simulink library "PTCL_lib"  (Simulink 7.5)
settings: Solver=ode45  StartTime=0.0  StopTime=10.0  RelTol=1e-3
values from neighbouring files (symbols this model uses):
  pPTCL_kw_DeltaTMAvlPwr_TAB = Simulink.Parameter    [PTCL_par.m]
  pPTCL_kw_MaxIDeltaTMAvlPwr_C = Simulink.Parameter    [PTCL_par.m]
  pPTCL_kw_MaxPIDeltaTMAvlPwr_C = Simulink.Parameter    [PTCL_par.m]
  pPTCL_kw_MinIDeltaTMAvlPwr_C = Simulink.Parameter    [PTCL_par.m]
  pPTCL_kw_MinPIDeltaTMAvlPwr_C = Simulink.Parameter    [PTCL_par.m]
  pPTCL_kw_MinTMAvailPwr_C = Simulink.Parameter    [PTCL_par.m]
  pPTCL_kw_PIActDeltaPwrThrsh_C = Simulink.Parameter    [PTCL_par.m]
  pPTCL_kw_PIActHysterDeltaPwr_C = Simulink.Parameter    [PTCL_par.m]
  pPTCL_Nm_MaxTrq_CUR = Simulink.Parameter    [PTCL_par.m]
  pPTCL_Nmps_DrvTrqLowrRateLim_C = Simulink.Parameter    [PTCL_par.m]
  pPTCL_Nmps_DrvTrqUpprRateLim_C = Simulink.Parameter    [PTCL_par.m]
  pPTCL_Nmps_RcpTrqLowrRateLim_C = Simulink.Parameter    [PTCL_par.m]
  pPTCL_Nmps_RcpTrqUpprRateLim_C = Simulink.Parameter    [PTCL_par.m]
  pPTCL_pct_DrvEffiFac_C = Simulink.Parameter    [PTCL_par.m]
  pPTCL_pct_Mot1EffLowrLim_C = Simulink.Parameter    [PTCL_par.m]
  pPTCL_pct_Mot1EffUpprLim_C = Simulink.Parameter    [PTCL_par.m]
  pPTCL_pct_RcpEffiFac_C = Simulink.Parameter    [PTCL_par.m]
  pPTCL_ratio_KI4DeltaTMAvlPwr_CUR = Simulink.Parameter    [PTCL_par.m]
  pPTCL_ratio_KP4DeltaTMAvlPwr_CUR = Simulink.Parameter    [PTCL_par.m]
  pPTCL_ratio_KwToW_M = Simulink.Parameter    [PTCL_par.m]
  pPTCL_ratio_MotSpdFiltFac_C = Simulink.Parameter    [PTCL_par.m]
  pPTCL_ratio_PwrToTrqFac_M = Simulink.Parameter    [PTCL_par.m]
  pPTCL_ratio_WToKw_M = Simulink.Parameter    [PTCL_par.m]
  pPTCL_rpm_RevLowrLim_C = Simulink.Parameter    [PTCL_par.m]
  pPTCL_rpm_RevUpprLim_C = Simulink.Parameter    [PTCL_par.m]
  pPTCL_rpm_TMSpd_TAB = Simulink.Parameter    [PTCL_par.m]
undefined symbols (not defined in the file or in its folder): p_single_Minus_M, p_single_Zero_M, pESPI_kmph_MinSpdSnsrThd_C, pMCI_m_TireDiam_C, pMCI_ratio_KmPerHrToMtrPerSec_C, pMCI_ratio_TrsmRat_C, pMCI_s_NoOfSec_C
libraries: BaseOperationLib_Browser x114, simulink x1
(part 1 of 2)
settings Model: Creator=wuaibin  LastModifiedBy=wuaibin

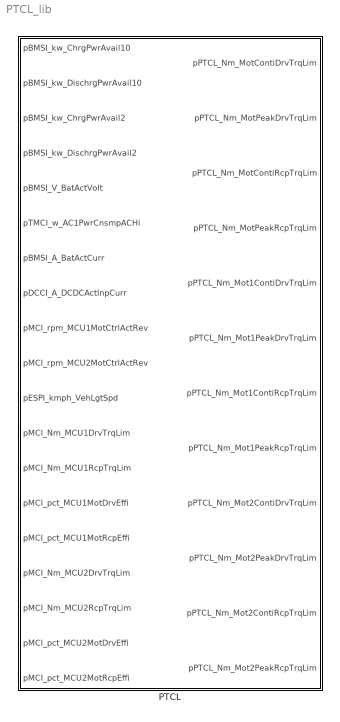
== system PTCL_lib ==
  PTCL : Subsystem  TreatAsAtomicUnit=on

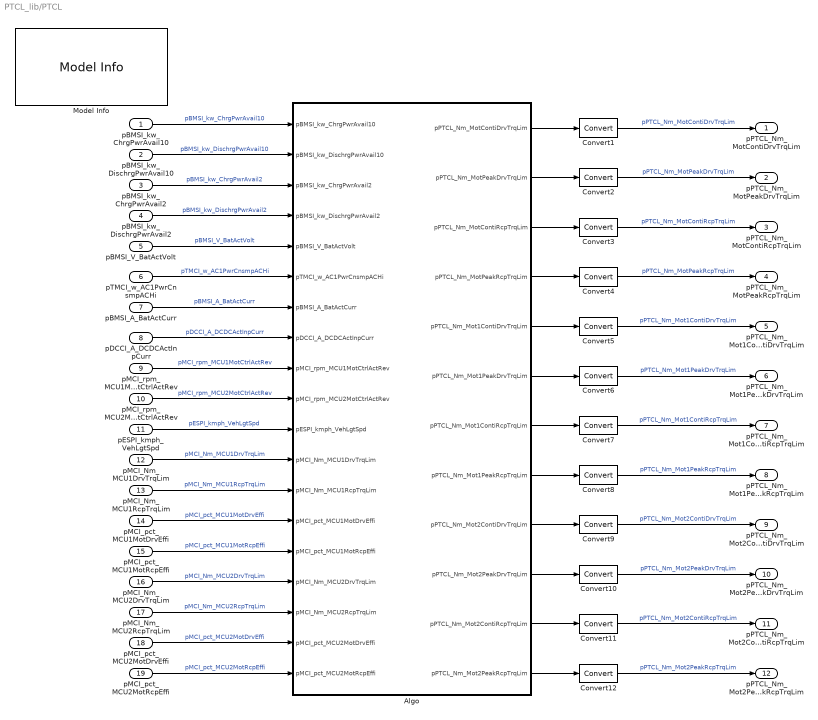
== system PTCL_lib/PTCL ==
  pBMSI_kw_ChrgPwrAvail10 : Inport
  pBMSI_kw_DischrgPwrAvail10 : Inport  Port=2
  pBMSI_kw_ChrgPwrAvail2 : Inport  Port=3
  pBMSI_kw_DischrgPwrAvail2 : Inport  Port=4
  pBMSI_V_BatActVolt : Inport  Port=5
  pTMCI_w_AC1PwrCnsmpACHi : Inport  Port=6
  pBMSI_A_BatActCurr : Inport  Port=7
  pDCCI_A_DCDCActInpCurr : Inport  Port=8
  pMCI_rpm_MCU1MotCtrlActRev : Inport  Port=9
  pMCI_rpm_MCU2MotCtrlActRev : Inport  Port=10
  pESPI_kmph_VehLgtSpd : Inport  Port=11
  pMCI_Nm_MCU1DrvTrqLim : Inport  Port=12
  pMCI_Nm_MCU1RcpTrqLim : Inport  Port=13
  pMCI_pct_MCU1MotDrvEffi : Inport  Port=14
  pMCI_pct_MCU1MotRcpEffi : Inport  Port=15
  pMCI_Nm_MCU2DrvTrqLim : Inport  Port=16
  pMCI_Nm_MCU2RcpTrqLim : Inport  Port=17
  pMCI_pct_MCU2MotDrvEffi : Inport  Port=18
  pMCI_pct_MCU2MotRcpEffi : Inport  Port=19
  Algo : Subsystem
  Convert{1..12} (12 alike) : DataTypeConversion  OutDataType=fixdt(1, 16)  OutScaling=2^0
  Model Info : simulink/Model-Wide Utilities/Model Info  SystemSampleTime=-1  InitialBlockCM=None  BlockCM=None  Frame=on  DisplayStringWithTags=Model Info\nCreated: %<Created>\nCreator: zhangqiang  HorizontalTextAlignment=Center  LeftAlignmentValue=0.5  SourceBlockDiagram=HQEV_HCU  TagMaxNumber=20
  pPTCL_Nm_MotContiDrvTrqLim : Outport
  pPTCL_Nm_MotPeakDrvTrqLim : Outport  Port=2
  pPTCL_Nm_MotContiRcpTrqLim : Outport  Port=3
  pPTCL_Nm_MotPeakRcpTrqLim : Outport  Port=4
  pPTCL_Nm_Mot1ContiDrvTrqLim : Outport  Port=5
  pPTCL_Nm_Mot1PeakDrvTrqLim : Outport  Port=6
  pPTCL_Nm_Mot1ContiRcpTrqLim : Outport  Port=7
  pPTCL_Nm_Mot1PeakRcpTrqLim : Outport  Port=8
  pPTCL_Nm_Mot2ContiDrvTrqLim : Outport  Port=9
  pPTCL_Nm_Mot2PeakDrvTrqLim : Outport  Port=10
  pPTCL_Nm_Mot2ContiRcpTrqLim : Outport  Port=11
  pPTCL_Nm_Mot2PeakRcpTrqLim : Outport  Port=12
  wires:
  pMCI_Nm_MCU2DrvTrqLim/1 -> Algo/16(pMCI_Nm_MCU2DrvTrqLim)  "pMCI_Nm_MCU2DrvTrqLim"
  pMCI_pct_MCU1MotRcpEffi/1 -> Algo/15(pMCI_pct_MCU1MotRcpEffi)  "pMCI_pct_MCU1MotRcpEffi"
  pMCI_pct_MCU1MotDrvEffi/1 -> Algo/14(pMCI_pct_MCU1MotDrvEffi)  "pMCI_pct_MCU1MotDrvEffi"
  pMCI_Nm_MCU1RcpTrqLim/1 -> Algo/13(pMCI_Nm_MCU1RcpTrqLim)  "pMCI_Nm_MCU1RcpTrqLim"
  pMCI_Nm_MCU1DrvTrqLim/1 -> Algo/12(pMCI_Nm_MCU1DrvTrqLim)  "pMCI_Nm_MCU1DrvTrqLim"
  pESPI_kmph_VehLgtSpd/1 -> Algo/11(pESPI_kmph_VehLgtSpd)  "pESPI_kmph_VehLgtSpd"
  pBMSI_kw_ChrgPwrAvail10/1 -> Algo/1(pBMSI_kw_ChrgPwrAvail10)  "pBMSI_kw_ChrgPwrAvail10"
  pBMSI_kw_DischrgPwrAvail10/1 -> Algo/2(pBMSI_kw_DischrgPwrAvail10)  "pBMSI_kw_DischrgPwrAvail10"
  pBMSI_kw_ChrgPwrAvail2/1 -> Algo/3(pBMSI_kw_ChrgPwrAvail2)  "pBMSI_kw_ChrgPwrAvail2"
  pBMSI_kw_DischrgPwrAvail2/1 -> Algo/4(pBMSI_kw_DischrgPwrAvail2)  "pBMSI_kw_DischrgPwrAvail2"
  pBMSI_V_BatActVolt/1 -> Algo/5(pBMSI_V_BatActVolt)  "pBMSI_V_BatActVolt"
  pTMCI_w_AC1PwrCnsmpACHi/1 -> Algo/6(pTMCI_w_AC1PwrCnsmpACHi)  "pTMCI_w_AC1PwrCnsmpACHi"
  pBMSI_A_BatActCurr/1 -> Algo/7(pBMSI_A_BatActCurr)  "pBMSI_A_BatActCurr"
  pDCCI_A_DCDCActInpCurr/1 -> Algo/8(pDCCI_A_DCDCActInpCurr)  "pDCCI_A_DCDCActInpCurr"
  pMCI_rpm_MCU1MotCtrlActRev/1 -> Algo/9(pMCI_rpm_MCU1MotCtrlActRev)  "pMCI_rpm_MCU1MotCtrlActRev"
  pMCI_rpm_MCU2MotCtrlActRev/1 -> Algo/10(pMCI_rpm_MCU2MotCtrlActRev)  "pMCI_rpm_MCU2MotCtrlActRev"
  Convert1/1 -> pPTCL_Nm_MotContiDrvTrqLim/1  "pPTCL_Nm_MotContiDrvTrqLim"
  Convert2/1 -> pPTCL_Nm_MotPeakDrvTrqLim/1  "pPTCL_Nm_MotPeakDrvTrqLim"
  Convert3/1 -> pPTCL_Nm_MotContiRcpTrqLim/1  "pPTCL_Nm_MotContiRcpTrqLim"
  Convert4/1 -> pPTCL_Nm_MotPeakRcpTrqLim/1  "pPTCL_Nm_MotPeakRcpTrqLim"
  Convert5/1 -> pPTCL_Nm_Mot1ContiDrvTrqLim/1  "pPTCL_Nm_Mot1ContiDrvTrqLim"
  pMCI_pct_MCU2MotRcpEffi/1 -> Algo/19(pMCI_pct_MCU2MotRcpEffi)  "pMCI_pct_MCU2MotRcpEffi"
  pMCI_pct_MCU2MotDrvEffi/1 -> Algo/18(pMCI_pct_MCU2MotDrvEffi)  "pMCI_pct_MCU2MotDrvEffi"
  pMCI_Nm_MCU2RcpTrqLim/1 -> Algo/17(pMCI_Nm_MCU2RcpTrqLim)  "pMCI_Nm_MCU2RcpTrqLim"
  Algo/1(pPTCL_Nm_MotContiDrvTrqLim) -> Convert1/1
  Algo/2(pPTCL_Nm_MotPeakDrvTrqLim) -> Convert2/1
  Algo/3(pPTCL_Nm_MotContiRcpTrqLim) -> Convert3/1
  Algo/4(pPTCL_Nm_MotPeakRcpTrqLim) -> Convert4/1
  Algo/5(pPTCL_Nm_Mot1ContiDrvTrqLim) -> Convert5/1
  Algo/6(pPTCL_Nm_Mot1PeakDrvTrqLim) -> Convert6/1
  Algo/7(pPTCL_Nm_Mot1ContiRcpTrqLim) -> Convert7/1
  Algo/8(pPTCL_Nm_Mot1PeakRcpTrqLim) -> Convert8/1
  Algo/9(pPTCL_Nm_Mot2ContiDrvTrqLim) -> Convert9/1
  Algo/10(pPTCL_Nm_Mot2PeakDrvTrqLim) -> Convert10/1
  Algo/12(pPTCL_Nm_Mot2PeakRcpTrqLim) -> Convert12/1
  Algo/11(pPTCL_Nm_Mot2ContiRcpTrqLim) -> Convert11/1
  Convert6/1 -> pPTCL_Nm_Mot1PeakDrvTrqLim/1  "pPTCL_Nm_Mot1PeakDrvTrqLim"
  Convert7/1 -> pPTCL_Nm_Mot1ContiRcpTrqLim/1  "pPTCL_Nm_Mot1ContiRcpTrqLim"
  Convert8/1 -> pPTCL_Nm_Mot1PeakRcpTrqLim/1  "pPTCL_Nm_Mot1PeakRcpTrqLim"
  Convert9/1 -> pPTCL_Nm_Mot2ContiDrvTrqLim/1  "pPTCL_Nm_Mot2ContiDrvTrqLim"
  Convert10/1 -> pPTCL_Nm_Mot2PeakDrvTrqLim/1  "pPTCL_Nm_Mot2PeakDrvTrqLim"
  Convert11/1 -> pPTCL_Nm_Mot2ContiRcpTrqLim/1  "pPTCL_Nm_Mot2ContiRcpTrqLim"
  Convert12/1 -> pPTCL_Nm_Mot2PeakRcpTrqLim/1  "pPTCL_Nm_Mot2PeakRcpTrqLim"

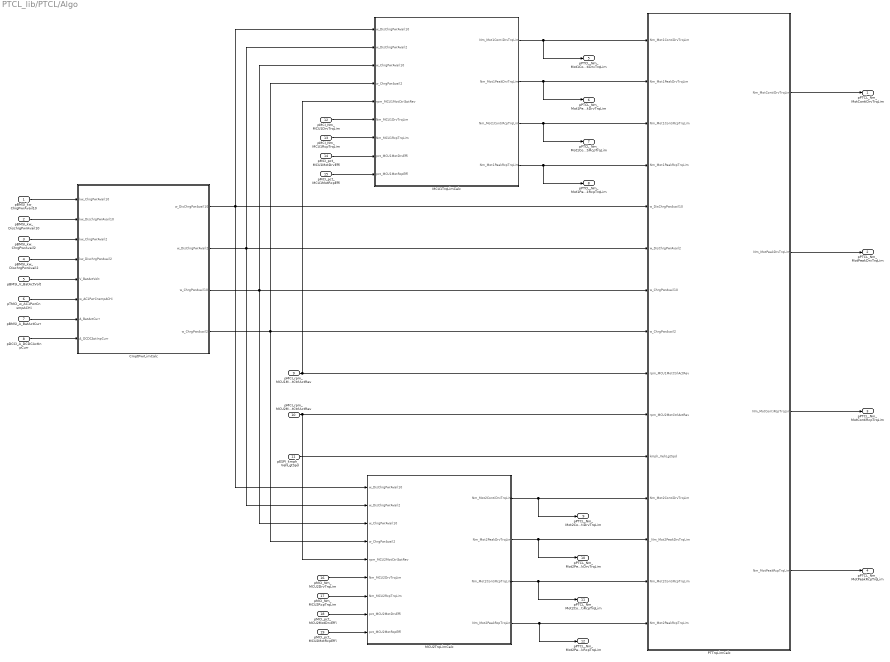
== system PTCL_lib/PTCL/Algo ==
  pBMSI_kw_ChrgPwrAvail10 : Inport
  pBMSI_kw_DischrgPwrAvail10 : Inport  Port=2
  pBMSI_kw_ChrgPwrAvail2 : Inport  Port=3
  pBMSI_kw_DischrgPwrAvail2 : Inport  Port=4
  pBMSI_V_BatActVolt : Inport  Port=5
  pTMCI_w_AC1PwrCnsmpACHi : Inport  Port=6
  pBMSI_A_BatActCurr : Inport  Port=7
  pDCCI_A_DCDCActInpCurr : Inport  Port=8
  pMCI_rpm_MCU1MotCtrlActRev : Inport  Port=9
  pMCI_rpm_MCU2MotCtrlActRev : Inport  Port=10
  pESPI_kmph_VehLgtSpd : Inport  Port=11
  pMCI_Nm_MCU1DrvTrqLim : Inport  Port=12
  pMCI_Nm_MCU1RcpTrqLim : Inport  Port=13
  pMCI_pct_MCU1MotDrvEffi : Inport  Port=14
  pMCI_pct_MCU1MotRcpEffi : Inport  Port=15
  pMCI_Nm_MCU2DrvTrqLim : Inport  Port=16
  pMCI_Nm_MCU2RcpTrqLim : Inport  Port=17
  pMCI_pct_MCU2MotDrvEffi : Inport  Port=18
  pMCI_pct_MCU2MotRcpEffi : Inport  Port=19
  CmptPwrLimCalc : Subsystem
  MCU1TrqLimCalc : Subsystem
  MCU2TrqLimCalc : Subsystem
  PTTrqLimCalc : Subsystem
  pPTCL_Nm_MotContiDrvTrqLim : Outport
  pPTCL_Nm_MotPeakDrvTrqLim : Outport  Port=2
  pPTCL_Nm_MotContiRcpTrqLim : Outport  Port=3
  pPTCL_Nm_MotPeakRcpTrqLim : Outport  Port=4
  pPTCL_Nm_Mot1ContiDrvTrqLim : Outport  Port=5
  pPTCL_Nm_Mot1PeakDrvTrqLim : Outport  Port=6
  pPTCL_Nm_Mot1ContiRcpTrqLim : Outport  Port=7
  pPTCL_Nm_Mot1PeakRcpTrqLim : Outport  Port=8
  pPTCL_Nm_Mot2ContiDrvTrqLim : Outport  Port=9
  pPTCL_Nm_Mot2PeakDrvTrqLim : Outport  Port=10
  pPTCL_Nm_Mot2ContiRcpTrqLim : Outport  Port=11
  pPTCL_Nm_Mot2PeakRcpTrqLim : Outport  Port=12
  wires:
  MCU1TrqLimCalc/1(Nm_Mot1ContiDrvTrqLim) -> pPTCL_Nm_Mot1ContiDrvTrqLim/1, PTTrqLimCalc/1(Nm_Mot1ContiDrvTrqLim)
  MCU1TrqLimCalc/2(Nm_Mot1PeakDrvTrqLim) -> pPTCL_Nm_Mot1PeakDrvTrqLim/1, PTTrqLimCalc/2(Nm_Mot1PeakDrvTrqLim)
  MCU1TrqLimCalc/3(Nm_Mot1ContiRcpTrqLim) -> pPTCL_Nm_Mot1ContiRcpTrqLim/1, PTTrqLimCalc/3(Nm_Mot1ContiRcpTrqLim)
  MCU1TrqLimCalc/4(Nm_Mot1PeakRcpTrqLim) -> pPTCL_Nm_Mot1PeakRcpTrqLim/1, PTTrqLimCalc/4(Nm_Mot1PeakRcpTrqLim)
  MCU2TrqLimCalc/1(Nm_Mot2ContiDrvTrqLim) -> PTTrqLimCalc/12(Nm_Mot2ContiDrvTrqLim), pPTCL_Nm_Mot2ContiDrvTrqLim/1
  MCU2TrqLimCalc/2(Nm_Mot2PeakDrvTrqLim) -> PTTrqLimCalc/13(_Nm_Mot2PeakDrvTrqLim), pPTCL_Nm_Mot2PeakDrvTrqLim/1
  MCU2TrqLimCalc/3(Nm_Mot2ContiRcpTrqLim) -> PTTrqLimCalc/14(Nm_Mot2ContiRcpTrqLim), pPTCL_Nm_Mot2ContiRcpTrqLim/1
  MCU2TrqLimCalc/4(Nm_Mot2PeakRcpTrqLim) -> PTTrqLimCalc/15(Nm_Mot2PeakRcpTrqLim), pPTCL_Nm_Mot2PeakRcpTrqLim/1
  PTTrqLimCalc/1(Nm_MotContiDrvTrqLim) -> pPTCL_Nm_MotContiDrvTrqLim/1
  PTTrqLimCalc/2(Nm_MotPeakDrvTrqLim) -> pPTCL_Nm_MotPeakDrvTrqLim/1
  PTTrqLimCalc/3(Nm_MotContiRcpTrqLim) -> pPTCL_Nm_MotContiRcpTrqLim/1
  PTTrqLimCalc/4(Nm_MotPeakRcpTrqLim) -> pPTCL_Nm_MotPeakRcpTrqLim/1
  CmptPwrLimCalc/1(w_DisChrgPwrAvail10) -> PTTrqLimCalc/5(w_DisChrgPwrAvail10), MCU2TrqLimCalc/1(w_DisChrgPwrAvail10), MCU1TrqLimCalc/1(w_DisChrgPwrAvail10)
  CmptPwrLimCalc/2(w_DisChrgPwrAvail2) -> PTTrqLimCalc/6(w_DisChrgPwrAvail2), MCU2TrqLimCalc/2(w_DisChrgPwrAvail2), MCU1TrqLimCalc/2(w_DisChrgPwrAvail2)
  CmptPwrLimCalc/3(w_ChrgPwrAvail10) -> PTTrqLimCalc/7(w_ChrgPwrAvail10), MCU1TrqLimCalc/3(w_ChrgPwrAvail10), MCU2TrqLimCalc/3(w_ChrgPwrAvail10)
  CmptPwrLimCalc/4(w_ChrgPwrAvail2) -> PTTrqLimCalc/8(w_ChrgPwrAvail2), MCU2TrqLimCalc/4(w_ChrgPwrAvail2), MCU1TrqLimCalc/4(w_ChrgPwrAvail2)
  pBMSI_kw_ChrgPwrAvail10/1 -> CmptPwrLimCalc/1(kw_ChrgPwrAvail10)
  pBMSI_kw_DischrgPwrAvail10/1 -> CmptPwrLimCalc/2(kw_DischrgPwrAvail10)
  pBMSI_kw_ChrgPwrAvail2/1 -> CmptPwrLimCalc/3(kw_ChrgPwrAvail2)
  pBMSI_kw_DischrgPwrAvail2/1 -> CmptPwrLimCalc/4(kw_DischrgPwrAvail2)
  pBMSI_V_BatActVolt/1 -> CmptPwrLimCalc/5(V_BatActVolt)
  pTMCI_w_AC1PwrCnsmpACHi/1 -> CmptPwrLimCalc/6(w_AC1PwrCnsmpACHi)
  pBMSI_A_BatActCurr/1 -> CmptPwrLimCalc/7(A_BatActCurr)
  pDCCI_A_DCDCActInpCurr/1 -> CmptPwrLimCalc/8(A_DCDCActInpCurr)
  pMCI_rpm_MCU1MotCtrlActRev/1 -> PTTrqLimCalc/9(rpm_MCU1MotCtrlActRev), MCU1TrqLimCalc/5(rpm_MCU1MotCtrlActRev)
  pMCI_rpm_MCU2MotCtrlActRev/1 -> PTTrqLimCalc/10(rpm_MCU2MotCtrlActRev), MCU2TrqLimCalc/5(rpm_MCU2MotCtrlActRev)
  pESPI_kmph_VehLgtSpd/1 -> PTTrqLimCalc/11(kmph_VehLgtSpd)
  pMCI_Nm_MCU1DrvTrqLim/1 -> MCU1TrqLimCalc/6(Nm_MCU1DrvTrqLim)
  pMCI_Nm_MCU1RcpTrqLim/1 -> MCU1TrqLimCalc/7(Nm_MCU1RcpTrqLim)
  pMCI_Nm_MCU2DrvTrqLim/1 -> MCU2TrqLimCalc/6(Nm_MCU2DrvTrqLim)
  pMCI_Nm_MCU2RcpTrqLim/1 -> MCU2TrqLimCalc/7(Nm_MCU2RcpTrqLim)
  pMCI_pct_MCU2MotDrvEffi/1 -> MCU2TrqLimCalc/8(pct_MCU2MotDrvEffi)
  pMCI_pct_MCU2MotRcpEffi/1 -> MCU2TrqLimCalc/9(pct_MCU2MotRcpEffi)
  pMCI_pct_MCU1MotDrvEffi/1 -> MCU1TrqLimCalc/8(pct_MCU1MotDrvEffi)
  pMCI_pct_MCU1MotRcpEffi/1 -> MCU1TrqLimCalc/9(pct_MCU1MotRcpEffi)

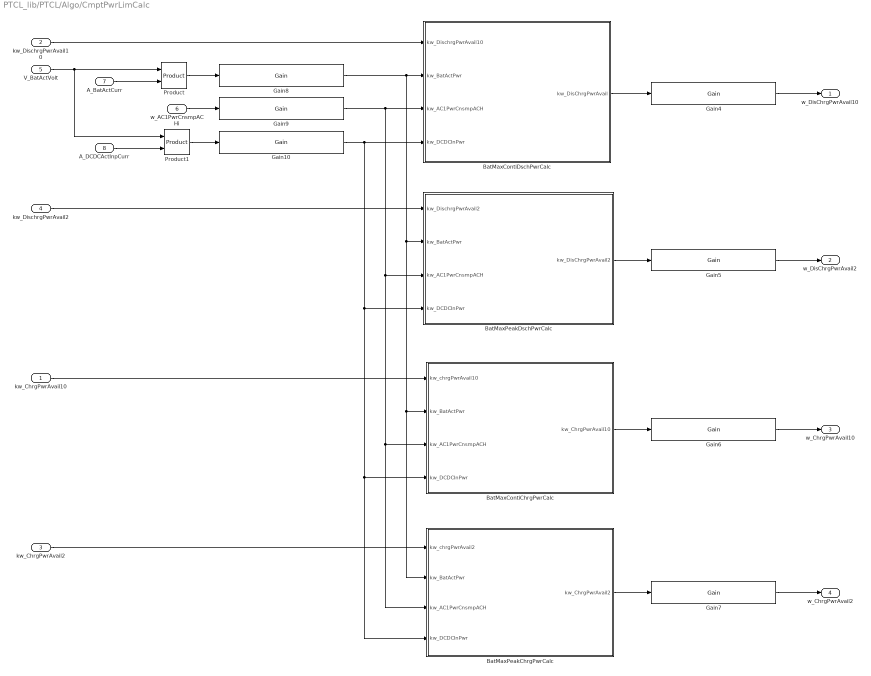
== system PTCL_lib/PTCL/Algo/CmptPwrLimCalc ==
  kw_ChrgPwrAvail10 : Inport
  kw_DischrgPwrAvail10 : Inport  Port=2
  kw_ChrgPwrAvail2 : Inport  Port=3
  kw_DischrgPwrAvail2 : Inport  Port=4
  V_BatActVolt : Inport  Port=5
  w_AC1PwrCnsmpACHi : Inport  Port=6  OutDataType=fixdt(1, 16)  OutScaling=2^0
  A_BatActCurr : Inport  Port=7
  A_DCDCActInpCurr : Inport  Port=8  OutDataType=fixdt(1, 16)  OutScaling=2^0
  BatMaxContiChrgPwrCalc : Subsystem
  BatMaxContiDschPwrCalc : Subsystem
  BatMaxPeakChrgPwrCalc : Subsystem
  BatMaxPeakDschPwrCalc : Subsystem
  Gain10 : BaseOperationLib_Browser/Math Operations Changed/Gain  Gain=pPTCL_ratio_WToKw_M  Multiplication=Element-wise(K.*u)  ParamMin=[]  ParamMax=[]  ParameterDataType=fixdt(1, 16)  ParameterScalingMode=Best Precision: Matrix-wise  ParameterScaling=2^0  ParamDataTypeStr=Inherit: Inherit from 'Gain'  OutMin=[]  OutMax=[]  OutDataType=fixdt(1, 16)  OutScaling=2^0  SaturateOnIntegerOverflow=on
  Gain{4..7} (4 alike) : BaseOperationLib_Browser/Math Operations Changed/Gain  Gain=pPTCL_ratio_KwToW_M  Multiplication=Element-wise(K.*u)  ParamMin=[]  ParamMax=[]  ParameterDataType=fixdt(1, 16)  ParameterScalingMode=Best Precision: Matrix-wise  ParameterScaling=2^0  ParamDataTypeStr=Inherit: Inherit from 'Gain'  OutMin=[]  OutMax=[]  OutDataType=fixdt(1, 16)  OutScaling=2^0  SaturateOnIntegerOverflow=on
  Gain8 : BaseOperationLib_Browser/Math Operations Changed/Gain  Gain=pPTCL_ratio_WToKw_M  Multiplication=Element-wise(K.*u)  ParamMin=[]  ParamMax=[]  ParameterDataType=fixdt(1, 16)  ParameterScalingMode=Best Precision: Matrix-wise  ParameterScaling=2^0  ParamDataTypeStr=Inherit: Inherit from 'Gain'  OutMin=[]  OutMax=[]  OutDataType=fixdt(1, 16)  OutScaling=2^0  SaturateOnIntegerOverflow=on
  Gain9 : BaseOperationLib_Browser/Math Operations Changed/Gain  Gain=pPTCL_ratio_WToKw_M  Multiplication=Element-wise(K.*u)  ParamMin=[]  ParamMax=[]  ParameterDataType=fixdt(1, 16)  ParameterScalingMode=Best Precision: Matrix-wise  ParameterScaling=2^0  ParamDataTypeStr=Inherit: Inherit from 'Gain'  OutMin=[]  OutMax=[]  OutDataType=fixdt(1, 16)  OutScaling=2^0  SaturateOnIntegerOverflow=on
  Product : BaseOperationLib_Browser/Math Operations Changed/Product  Inputs=2  Multiplication=Element-wise(.*)  OutMin=[]  OutMax=[]  OutDataType=fixdt(1,16,0)  OutScaling=[]  OutDataTypeStr=Inherit: Inherit via back propagation  RndMeth=Zero  SaturateOnIntegerOverflow=on
  Product1 : BaseOperationLib_Browser/Math Operations Changed/Product  Inputs=2  Multiplication=Element-wise(.*)  OutMin=[]  OutMax=[]  OutDataType=fixdt(1,16,0)  OutScaling=[]  OutDataTypeStr=Inherit: Inherit via back propagation  RndMeth=Zero  SaturateOnIntegerOverflow=on
  w_DisChrgPwrAvail10 : Outport  OutDataType=fixdt(1, 16)  OutScaling=2^0
  w_DisChrgPwrAvail2 : Outport  Port=2  OutDataType=fixdt(1, 16)  OutScaling=2^0
  w_ChrgPwrAvail10 : Outport  Port=3  OutDataType=fixdt(1, 16)  OutScaling=2^0
  w_ChrgPwrAvail2 : Outport  Port=4  OutDataType=fixdt(1, 16)  OutScaling=2^0
  wires:
  V_BatActVolt/1 -> Product/1, Product1/1
  A_BatActCurr/1 -> Product/2
  A_DCDCActInpCurr/1 -> Product1/2
  kw_DischrgPwrAvail10/1 -> BatMaxContiDschPwrCalc/1(kw_DischrgPwrAvail10)
  Product/1 -> Gain8/1
  w_AC1PwrCnsmpACHi/1 -> Gain9/1
  Product1/1 -> Gain10/1
  kw_DischrgPwrAvail2/1 -> BatMaxPeakDschPwrCalc/1(kw_DischrgPwrAvail2)
  kw_ChrgPwrAvail10/1 -> BatMaxContiChrgPwrCalc/1(kw_chrgPwrAvail10)
  kw_ChrgPwrAvail2/1 -> BatMaxPeakChrgPwrCalc/1(kw_chrgPwrAvail2)
  BatMaxPeakChrgPwrCalc/1(kw_ChrgPwrAvail2) -> Gain7/1
  BatMaxContiChrgPwrCalc/1(kw_ChrgPwrAvail10) -> Gain6/1
  BatMaxPeakDschPwrCalc/1(kw_DisChrgPwrAvail2) -> Gain5/1
  BatMaxContiDschPwrCalc/1(kw_DisChrgPwrAvail) -> Gain4/1
  Gain4/1 -> w_DisChrgPwrAvail10/1
  Gain5/1 -> w_DisChrgPwrAvail2/1
  Gain6/1 -> w_ChrgPwrAvail10/1
  Gain7/1 -> w_ChrgPwrAvail2/1
  Gain8/1 -> BatMaxContiDschPwrCalc/2(kw_BatActPwr), BatMaxPeakDschPwrCalc/2(kw_BatActPwr), BatMaxContiChrgPwrCalc/2(kw_BatActPwr), BatMaxPeakChrgPwrCalc/2(kw_BatActPwr)
  Gain9/1 -> BatMaxContiDschPwrCalc/3(kw_AC1PwrCnsmpACH), BatMaxPeakDschPwrCalc/3(kw_AC1PwrCnsmpACH), BatMaxContiChrgPwrCalc/3(kw_AC1PwrCnsmpACH), BatMaxPeakChrgPwrCalc/3(kw_AC1PwrCnsmpACH)
  Gain10/1 -> BatMaxContiDschPwrCalc/4(kw_DCDCInPwr), BatMaxPeakDschPwrCalc/4(kw_DCDCInPwr), BatMaxContiChrgPwrCalc/4(kw_DCDCInPwr), BatMaxPeakChrgPwrCalc/4(kw_DCDCInPwr)

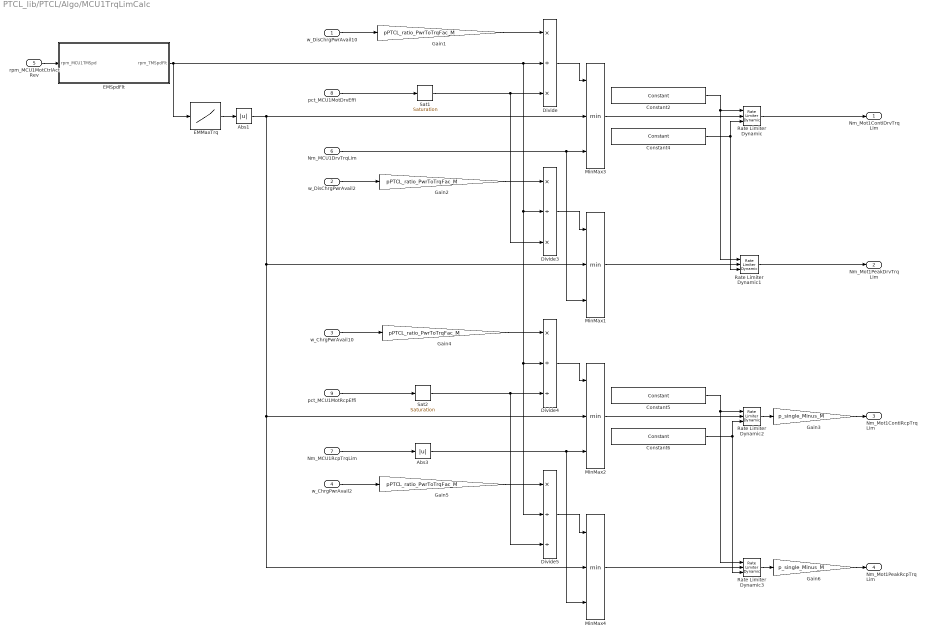
== system PTCL_lib/PTCL/Algo/MCU1TrqLimCalc ==
  w_DisChrgPwrAvail10 : Inport
  w_DisChrgPwrAvail2 : Inport  Port=2
  w_ChrgPwrAvail10 : Inport  Port=3
  w_ChrgPwrAvail2 : Inport  Port=4
  rpm_MCU1MotCtrlActRev : Inport  Port=5
  Nm_MCU1DrvTrqLim : Inport  Port=6
  Nm_MCU1RcpTrqLim : Inport  Port=7
  pct_MCU1MotDrvEffi : Inport  Port=8
  pct_MCU1MotRcpEffi : Inport  Port=9
  Abs1 : Abs  SaturateOnIntegerOverflow=on
      mask Display: patch([0 1 1 1 .75], [1 1 0 .75 1], [0 1 0]);
  Abs3 : Abs  SaturateOnIntegerOverflow=on
      mask Display: patch([0 1 1 1 .75], [1 1 0 .75 1], [0 1 0]);
  Constant2 : BaseOperationLib_Browser/Sources&Sinks/Constant  Value=pPTCL_Nmps_DrvTrqUpprRateLim_C  OutMin=[]  OutMax=[]  OutDataType=fixdt(1, 16)  ConRadixGroup=Use specified scaling  OutScaling=2^0  OutDataTypeStr=Inherit: Inherit from 'Constant value'
  Constant4 : BaseOperationLib_Browser/Sources&Sinks/Constant  Value=pPTCL_Nmps_DrvTrqLowrRateLim_C  OutMin=[]  OutMax=[]  OutDataType=fixdt(1, 16)  ConRadixGroup=Use specified scaling  OutScaling=2^0  OutDataTypeStr=Inherit: Inherit from 'Constant value'
  Constant5 : BaseOperationLib_Browser/Sources&Sinks/Constant  Value=pPTCL_Nmps_RcpTrqUpprRateLim_C  OutMin=[]  OutMax=[]  OutDataType=fixdt(1, 16)  ConRadixGroup=Use specified scaling  OutScaling=2^0  OutDataTypeStr=Inherit: Inherit from 'Constant value'
  Constant6 : BaseOperationLib_Browser/Sources&Sinks/Constant  Value=pPTCL_Nmps_RcpTrqLowrRateLim_C  OutMin=[]  OutMax=[]  OutDataType=fixdt(1, 16)  ConRadixGroup=Use specified scaling  OutScaling=2^0  OutDataTypeStr=Inherit: Inherit from 'Constant value'
  Divide : Product  Inputs=*/*  OutDataTypeStr=Inherit: Inherit via back propagation  SaturateOnIntegerOverflow=on
      mask Display: patch([0 1 1 1 .75], [1 1 0 .75 1], [0 1 0]);
  Divide3 : Product  Inputs=*/*  OutDataTypeStr=Inherit: Inherit via back propagation  SaturateOnIntegerOverflow=on
      mask Display: patch([0 1 1 1 .75], [1 1 0 .75 1], [0 1 0]);
  Divide4 : Product  Inputs=*//  OutDataTypeStr=Inherit: Inherit via back propagation  SaturateOnIntegerOverflow=on
      mask Display: patch([0 1 1 1 .75], [1 1 0 .75 1], [0 1 0]);
  Divide5 : Product  Inputs=*//  OutDataTypeStr=Inherit: Inherit via back propagation  SaturateOnIntegerOverflow=on
      mask Display: patch([0 1 1 1 .75], [1 1 0 .75 1], [0 1 0]);
  EMMaxTrq : Lookup  InputValues=pPTCL_rpm_TMSpd_TAB  Table=pPTCL_Nm_MaxTrq_CUR  LookUpMeth=Interpolation-Use End Values  OutDataTypeStr=Inherit: Inherit via back propagation  SaturateOnIntegerOverflow=on
      settings: AttributesFormatString=X:%<InputValues>\nTAB:%<Table>
      mask Display: patch([0 1 1 1 .75], [1 1 0 .75 1], [0 1 0]);
  EMSpdFlt : Subsystem
  Gain{1..2,4..5} (4 alike) : Gain  Gain=pPTCL_ratio_PwrToTrqFac_M  SaturateOnIntegerOverflow=on  OutDataTypeStr=Inherit: Same as input
      mask Display: patch([0 1 1 1 .75], [1 1 0 .75 1], [0 1 0]);
  Gain3 : Gain  Gain=p_single_Minus_M  SaturateOnIntegerOverflow=on  OutDataTypeStr=Inherit: Same as input
      mask Display: patch([0 1 1 1 .75], [1 1 0 .75 1], [0 1 0]);
  Gain6 : Gain  Gain=p_single_Minus_M  SaturateOnIntegerOverflow=on  OutDataTypeStr=Inherit: Same as input
      mask Display: patch([0 1 1 1 .75], [1 1 0 .75 1], [0 1 0]);
  MinMax{1..4} (4 alike) : MinMax  Inputs=3  SaturateOnIntegerOverflow=on  InputSameDT=on
      mask Display: patch([0 1 1 1 .75], [1 1 0 .75 1], [0 1 0]);
  Rate Limiter Dynamic{,1..3} (4 alike) : BaseOperationLib_Browser/Discontinuities Unchanged/Rate Limiter Dynamic  SystemSampleTime=-1
  Sat1 : BaseOperationLib_Browser/Discontinuities Unchanged/Saturation  UpperLimit=pPTCL_pct_Mot1EffUpprLim_C  LowerLimit=pPTCL_pct_Mot1EffLowrLim_C  OutMin=[]  OutMax=[]  OutDataType=fixdt(1, 16)  OutScaling=2^0  OutDataTypeStr=Inherit: Inherit via back propagation
      settings: AttributesFormatString=ULim:%<UpperLimit>\nLLim:%<LowerLimit>
  Sat2 : BaseOperationLib_Browser/Discontinuities Unchanged/Saturation  UpperLimit=pPTCL_pct_Mot1EffUpprLim_C  LowerLimit=pPTCL_pct_Mot1EffLowrLim_C  OutMin=[]  OutMax=[]  OutDataType=fixdt(1, 16)  OutScaling=2^0  OutDataTypeStr=Inherit: Inherit via back propagation
      settings: AttributesFormatString=ULim:%<UpperLimit>\nLLim:%<LowerLimit>
  Nm_Mot1ContiDrvTrqLim : Outport
  Nm_Mot1PeakDrvTrqLim : Outport  Port=2
  Nm_Mot1ContiRcpTrqLim : Outport  Port=3
  Nm_Mot1PeakRcpTrqLim : Outport  Port=4
  wires:
  Abs3/1 -> MinMax4/3, MinMax2/3
  Nm_MCU1DrvTrqLim/1 -> MinMax1/3, MinMax3/3
  Nm_MCU1RcpTrqLim/1 -> Abs3/1
  Abs1/1 -> MinMax4/2, MinMax2/2, MinMax1/2, MinMax3/2
  EMMaxTrq/1 -> Abs1/1
  w_DisChrgPwrAvail10/1 -> Gain1/1
  rpm_MCU1MotCtrlActRev/1 -> EMSpdFlt/1(rpm_MCU1TMSpd)
  Divide/1 -> MinMax3/1
  Sat1/1 -> Divide/3, Divide3/3
  pct_MCU1MotDrvEffi/1 -> Sat1/1
  Gain1/1 -> Divide/1
  w_DisChrgPwrAvail2/1 -> Gain2/1
  Gain2/1 -> Divide3/1
  Divide3/1 -> MinMax1/1
  w_ChrgPwrAvail10/1 -> Gain4/1
  Divide4/1 -> MinMax2/1
  pct_MCU1MotRcpEffi/1 -> Sat2/1
  Gain4/1 -> Divide4/1
  w_ChrgPwrAvail2/1 -> Gain5/1
  Gain5/1 -> Divide5/1
  Divide5/1 -> MinMax4/1
  EMSpdFlt/1(rpm_TMSpdFlt) -> Divide/2, Divide4/2, Divide5/2, Divide3/2, EMMaxTrq/1
  Rate Limiter Dynamic/1 -> Nm_Mot1ContiDrvTrqLim/1
  MinMax3/1 -> Rate Limiter Dynamic/2
  Rate Limiter Dynamic1/1 -> Nm_Mot1PeakDrvTrqLim/1
  MinMax1/1 -> Rate Limiter Dynamic1/2
  Rate Limiter Dynamic2/1 -> Gain3/1
  Rate Limiter Dynamic3/1 -> Gain6/1
  Constant2/1 -> Rate Limiter Dynamic/1, Rate Limiter Dynamic1/1
  Constant4/1 -> Rate Limiter Dynamic/3, Rate Limiter Dynamic1/3
  Constant5/1 -> Rate Limiter Dynamic2/1, Rate Limiter Dynamic3/1
  Constant6/1 -> Rate Limiter Dynamic2/3, Rate Limiter Dynamic3/3
  MinMax2/1 -> Rate Limiter Dynamic2/2
  MinMax4/1 -> Rate Limiter Dynamic3/2
  Gain3/1 -> Nm_Mot1ContiRcpTrqLim/1
  Gain6/1 -> Nm_Mot1PeakRcpTrqLim/1
  Sat2/1 -> Divide5/3, Divide4/3

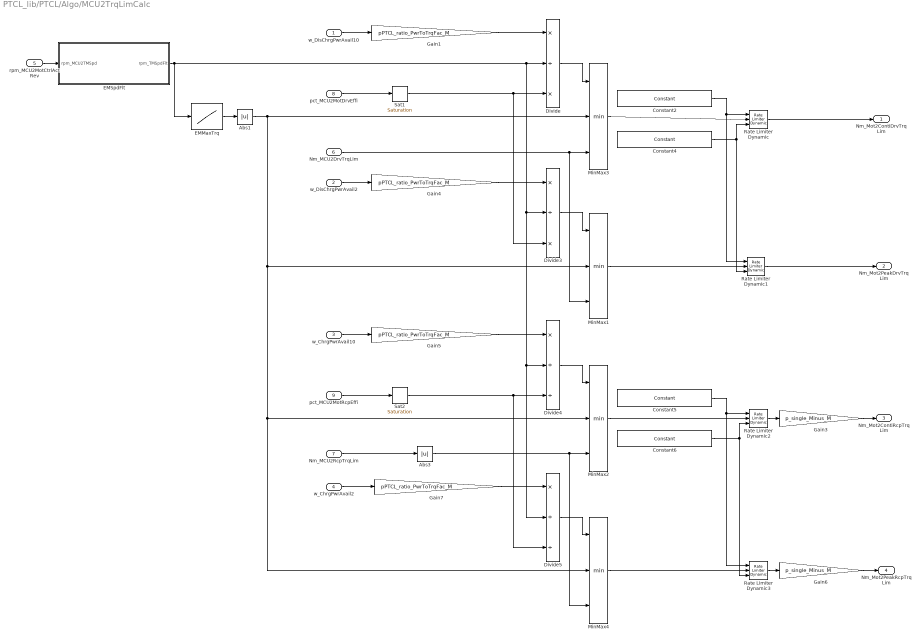
== system PTCL_lib/PTCL/Algo/MCU2TrqLimCalc ==
  w_DisChrgPwrAvail10 : Inport
  w_DisChrgPwrAvail2 : Inport  Port=2
  w_ChrgPwrAvail10 : Inport  Port=3
  w_ChrgPwrAvail2 : Inport  Port=4
  rpm_MCU2MotCtrlActRev : Inport  Port=5
  Nm_MCU2DrvTrqLim : Inport  Port=6
  Nm_MCU2RcpTrqLim : Inport  Port=7
  pct_MCU2MotDrvEffi : Inport  Port=8
  pct_MCU2MotRcpEffi : Inport  Port=9
  Abs1 : Abs  SaturateOnIntegerOverflow=on
      mask Display: patch([0 1 1 1 .75], [1 1 0 .75 1], [0 1 0]);
  Abs3 : Abs  SaturateOnIntegerOverflow=on
      mask Display: patch([0 1 1 1 .75], [1 1 0 .75 1], [0 1 0]);
  Constant2 : BaseOperationLib_Browser/Sources&Sinks/Constant  Value=pPTCL_Nmps_DrvTrqUpprRateLim_C  OutMin=[]  OutMax=[]  OutDataType=fixdt(1, 16)  ConRadixGroup=Use specified scaling  OutScaling=2^0  OutDataTypeStr=Inherit: Inherit from 'Constant value'
  Constant4 : BaseOperationLib_Browser/Sources&Sinks/Constant  Value=pPTCL_Nmps_DrvTrqLowrRateLim_C  OutMin=[]  OutMax=[]  OutDataType=fixdt(1, 16)  ConRadixGroup=Use specified scaling  OutScaling=2^0  OutDataTypeStr=Inherit: Inherit from 'Constant value'
  Constant5 : BaseOperationLib_Browser/Sources&Sinks/Constant  Value=pPTCL_Nmps_RcpTrqUpprRateLim_C  OutMin=[]  OutMax=[]  OutDataType=fixdt(1, 16)  ConRadixGroup=Use specified scaling  OutScaling=2^0  OutDataTypeStr=Inherit: Inherit from 'Constant value'
  Constant6 : BaseOperationLib_Browser/Sources&Sinks/Constant  Value=pPTCL_Nmps_RcpTrqLowrRateLim_C  OutMin=[]  OutMax=[]  OutDataType=fixdt(1, 16)  ConRadixGroup=Use specified scaling  OutScaling=2^0  OutDataTypeStr=Inherit: Inherit from 'Constant value'
  Divide : Product  Inputs=*/*  OutDataTypeStr=Inherit: Inherit via back propagation  SaturateOnIntegerOverflow=on
      mask Display: patch([0 1 1 1 .75], [1 1 0 .75 1], [0 1 0]);
  Divide3 : Product  Inputs=*/*  OutDataTypeStr=Inherit: Inherit via back propagation  SaturateOnIntegerOverflow=on
      mask Display: patch([0 1 1 1 .75], [1 1 0 .75 1], [0 1 0]);
  Divide4 : Product  Inputs=*//  OutDataTypeStr=Inherit: Inherit via back propagation  SaturateOnIntegerOverflow=on
      mask Display: patch([0 1 1 1 .75], [1 1 0 .75 1], [0 1 0]);
  Divide5 : Product  Inputs=*//  OutDataTypeStr=Inherit: Inherit via back propagation  SaturateOnIntegerOverflow=on
      mask Display: patch([0 1 1 1 .75], [1 1 0 .75 1], [0 1 0]);
  EMMaxTrq : Lookup  InputValues=pPTCL_rpm_TMSpd_TAB  Table=pPTCL_Nm_MaxTrq_CUR  LookUpMeth=Interpolation-Use End Values  OutDataTypeStr=Inherit: Inherit via back propagation  SaturateOnIntegerOverflow=on
      settings: AttributesFormatString=X:%<InputValues>\nTAB:%<Table>
      mask Display: patch([0 1 1 1 .75], [1 1 0 .75 1], [0 1 0]);
  EMSpdFlt : Subsystem
  Gain{1,4..5,7} (4 alike) : Gain  Gain=pPTCL_ratio_PwrToTrqFac_M  SaturateOnIntegerOverflow=on  OutDataTypeStr=Inherit: Same as input
      mask Display: patch([0 1 1 1 .75], [1 1 0 .75 1], [0 1 0]);
  Gain3 : Gain  Gain=p_single_Minus_M  SaturateOnIntegerOverflow=on  OutDataTypeStr=Inherit: Same as input
      mask Display: patch([0 1 1 1 .75], [1 1 0 .75 1], [0 1 0]);
  Gain6 : Gain  Gain=p_single_Minus_M  SaturateOnIntegerOverflow=on  OutDataTypeStr=Inherit: Same as input
      mask Display: patch([0 1 1 1 .75], [1 1 0 .75 1], [0 1 0]);
  MinMax{1..4} (4 alike) : MinMax  Inputs=3  SaturateOnIntegerOverflow=on  InputSameDT=on
      mask Display: patch([0 1 1 1 .75], [1 1 0 .75 1], [0 1 0]);
  Rate Limiter Dynamic{,1..3} (4 alike) : BaseOperationLib_Browser/Discontinuities Unchanged/Rate Limiter Dynamic  SystemSampleTime=-1
  Sat1 : BaseOperationLib_Browser/Discontinuities Unchanged/Saturation  UpperLimit=pPTCL_pct_Mot1EffUpprLim_C  LowerLimit=pPTCL_pct_Mot1EffLowrLim_C  OutMin=[]  OutMax=[]  OutDataType=fixdt(1, 16)  OutScaling=2^0  OutDataTypeStr=Inherit: Inherit via back propagation
      settings: AttributesFormatString=ULim:%<UpperLimit>\nLLim:%<LowerLimit>
  Sat2 : BaseOperationLib_Browser/Discontinuities Unchanged/Saturation  UpperLimit=pPTCL_pct_Mot1EffUpprLim_C  LowerLimit=pPTCL_pct_Mot1EffLowrLim_C  OutMin=[]  OutMax=[]  OutDataType=fixdt(1, 16)  OutScaling=2^0  OutDataTypeStr=Inherit: Inherit via back propagation
      settings: AttributesFormatString=ULim:%<UpperLimit>\nLLim:%<LowerLimit>
  Nm_Mot2ContiDrvTrqLim : Outport
  Nm_Mot2PeakDrvTrqLim : Outport  Port=2
  Nm_Mot2ContiRcpTrqLim : Outport  Port=3
  Nm_Mot2PeakRcpTrqLim : Outport  Port=4
  wires:
  EMSpdFlt/1(rpm_TMSpdFlt) -> EMMaxTrq/1, Divide3/2, Divide5/2, Divide4/2, Divide/2
  Divide5/1 -> MinMax4/1
  Gain7/1 -> Divide5/1
  w_ChrgPwrAvail2/1 -> Gain7/1
  Gain5/1 -> Divide4/1
  pct_MCU2MotRcpEffi/1 -> Sat2/1
  Sat2/1 -> Divide4/3, Divide5/3
  Divide4/1 -> MinMax2/1
  w_ChrgPwrAvail10/1 -> Gain5/1
  Divide3/1 -> MinMax1/1
  Gain4/1 -> Divide3/1
  w_DisChrgPwrAvail2/1 -> Gain4/1
  Gain1/1 -> Divide/1
  pct_MCU2MotDrvEffi/1 -> Sat1/1
  Sat1/1 -> Divide3/3, Divide/3
  Divide/1 -> MinMax3/1
  rpm_MCU2MotCtrlActRev/1 -> EMSpdFlt/1(rpm_MCU2TMSpd)
  w_DisChrgPwrAvail10/1 -> Gain1/1
  EMMaxTrq/1 -> Abs1/1
  Abs1/1 -> MinMax3/2, MinMax1/2, MinMax2/2, MinMax4/2
  Nm_MCU2RcpTrqLim/1 -> Abs3/1
  Nm_MCU2DrvTrqLim/1 -> MinMax3/3, MinMax1/3
  Abs3/1 -> MinMax2/3, MinMax4/3
  Rate Limiter Dynamic/1 -> Nm_Mot2ContiDrvTrqLim/1
  MinMax3/1 -> Rate Limiter Dynamic/2
  Rate Limiter Dynamic1/1 -> Nm_Mot2PeakDrvTrqLim/1
  MinMax1/1 -> Rate Limiter Dynamic1/2
  Rate Limiter Dynamic2/1 -> Gain3/1
  MinMax2/1 -> Rate Limiter Dynamic2/2
  Rate Limiter Dynamic3/1 -> Gain6/1
  MinMax4/1 -> Rate Limiter Dynamic3/2
  Constant2/1 -> Rate Limiter Dynamic/1, Rate Limiter Dynamic1/1
  Constant4/1 -> Rate Limiter Dynamic/3, Rate Limiter Dynamic1/3
  Constant5/1 -> Rate Limiter Dynamic2/1, Rate Limiter Dynamic3/1
  Constant6/1 -> Rate Limiter Dynamic2/3, Rate Limiter Dynamic3/3
  Gain3/1 -> Nm_Mot2ContiRcpTrqLim/1
  Gain6/1 -> Nm_Mot2PeakRcpTrqLim/1

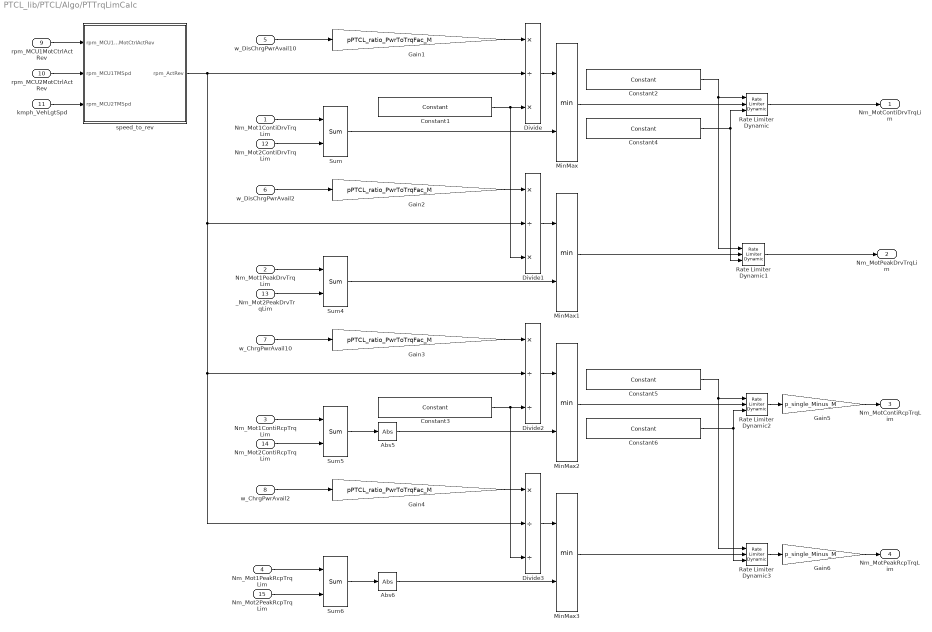
== system PTCL_lib/PTCL/Algo/PTTrqLimCalc ==
  Nm_Mot1ContiDrvTrqLim : Inport
  Nm_Mot1PeakDrvTrqLim : Inport  Port=2
  Nm_Mot1ContiRcpTrqLim : Inport  Port=3
  Nm_Mot1PeakRcpTrqLim : Inport  Port=4
  w_DisChrgPwrAvail10 : Inport  Port=5
  w_DisChrgPwrAvail2 : Inport  Port=6
  w_ChrgPwrAvail10 : Inport  Port=7
  w_ChrgPwrAvail2 : Inport  Port=8
  rpm_MCU1MotCtrlActRev : Inport  Port=9  OutDataType=fixdt(1, 16)  OutScaling=2^0
  rpm_MCU2MotCtrlActRev : Inport  Port=10  OutDataType=fixdt(1, 16)  OutScaling=2^0
  kmph_VehLgtSpd : Inport  Port=11  OutDataType=fixdt(1, 16)  OutScaling=2^0
  Nm_Mot2ContiDrvTrqLim : Inport  Port=12
  _Nm_Mot2PeakDrvTrqLim : Inport  Port=13
  Nm_Mot2ContiRcpTrqLim : Inport  Port=14
  Nm_Mot2PeakRcpTrqLim : Inport  Port=15
  Abs5 : BaseOperationLib_Browser/Math Operations Changed/Abs  OutMax=[]  OutDataType=fixdt(1, 16)  OutScaling=2^0
  Abs6 : BaseOperationLib_Browser/Math Operations Changed/Abs  OutMax=[]  OutDataType=fixdt(1, 16)  OutScaling=2^0
  Constant1 : BaseOperationLib_Browser/Sources&Sinks/Constant  Value=pPTCL_pct_DrvEffiFac_C  OutMin=[]  OutMax=[]  OutDataType=fixdt(1, 16)  ConRadixGroup=Use specified scaling  OutScaling=2^0  OutDataTypeStr=Inherit: Inherit from 'Constant value'
  Constant2 : BaseOperationLib_Browser/Sources&Sinks/Constant  Value=pPTCL_Nmps_DrvTrqUpprRateLim_C  OutMin=[]  OutMax=[]  OutDataType=fixdt(1, 16)  ConRadixGroup=Use specified scaling  OutScaling=2^0  OutDataTypeStr=Inherit: Inherit from 'Constant value'
  Constant3 : BaseOperationLib_Browser/Sources&Sinks/Constant  Value=pPTCL_pct_RcpEffiFac_C  OutMin=[]  OutMax=[]  OutDataType=fixdt(1, 16)  ConRadixGroup=Use specified scaling  OutScaling=2^0  OutDataTypeStr=Inherit: Inherit from 'Constant value'
  Constant4 : BaseOperationLib_Browser/Sources&Sinks/Constant  Value=pPTCL_Nmps_DrvTrqLowrRateLim_C  OutMin=[]  OutMax=[]  OutDataType=fixdt(1, 16)  ConRadixGroup=Use specified scaling  OutScaling=2^0  OutDataTypeStr=Inherit: Inherit from 'Constant value'
  Constant5 : BaseOperationLib_Browser/Sources&Sinks/Constant  Value=pPTCL_Nmps_RcpTrqUpprRateLim_C  OutMin=[]  OutMax=[]  OutDataType=fixdt(1, 16)  ConRadixGroup=Use specified scaling  OutScaling=2^0  OutDataTypeStr=Inherit: Inherit from 'Constant value'
  Constant6 : BaseOperationLib_Browser/Sources&Sinks/Constant  Value=pPTCL_Nmps_RcpTrqLowrRateLim_C  OutMin=[]  OutMax=[]  OutDataType=fixdt(1, 16)  ConRadixGroup=Use specified scaling  OutScaling=2^0  OutDataTypeStr=Inherit: Inherit from 'Constant value'
  Divide : Product  Inputs=*/*  OutDataTypeStr=Inherit: Inherit via back propagation  SaturateOnIntegerOverflow=on
      mask Display: patch([0 1 1 1 .75], [1 1 0 .75 1], [0 1 0]);
  Divide1 : Product  Inputs=*/*  OutDataTypeStr=Inherit: Inherit via back propagation  SaturateOnIntegerOverflow=on
      mask Display: patch([0 1 1 1 .75], [1 1 0 .75 1], [0 1 0]);
  Divide2 : Product  Inputs=*//  OutDataTypeStr=Inherit: Inherit via back propagation  SaturateOnIntegerOverflow=on
      mask Display: patch([0 1 1 1 .75], [1 1 0 .75 1], [0 1 0]);
  Divide3 : Product  Inputs=*//  OutDataTypeStr=Inherit: Inherit via back propagation  SaturateOnIntegerOverflow=on
      mask Display: patch([0 1 1 1 .75], [1 1 0 .75 1], [0 1 0]);
  Gain{1..4} (4 alike) : Gain  Gain=pPTCL_ratio_PwrToTrqFac_M  SaturateOnIntegerOverflow=on  OutDataTypeStr=Inherit: Same as input
      mask Display: patch([0 1 1 1 .75], [1 1 0 .75 1], [0 1 0]);
  Gain5 : Gain  Gain=p_single_Minus_M  SaturateOnIntegerOverflow=on  OutDataTypeStr=Inherit: Same as input
      mask Display: patch([0 1 1 1 .75], [1 1 0 .75 1], [0 1 0]);
  Gain6 : Gain  Gain=p_single_Minus_M  SaturateOnIntegerOverflow=on  OutDataTypeStr=Inherit: Same as input
      mask Display: patch([0 1 1 1 .75], [1 1 0 .75 1], [0 1 0]);
  MinMax{,1..3} (4 alike) : MinMax  Inputs=2  SaturateOnIntegerOverflow=on  InputSameDT=on
      mask Display: patch([0 1 1 1 .75], [1 1 0 .75 1], [0 1 0]);
  Rate Limiter Dynamic{,1..3} (4 alike) : BaseOperationLib_Browser/Discontinuities Unchanged/Rate Limiter Dynamic  SystemSampleTime=-1
  Sum{,4..6} (4 alike) : BaseOperationLib_Browser/Math Operations Changed/Sum  Inputs=++  InputSameDT=on  OutMin=[]  OutMax=[]  OutDataType=fixdt(1, 16)  OutScaling=2^0  SaturateOnIntegerOverflow=on
  speed_to_rev : Subsystem
  Nm_MotContiDrvTrqLim : Outport
  Nm_MotPeakDrvTrqLim : Outport  Port=2
  Nm_MotContiRcpTrqLim : Outport  Port=3
  Nm_MotPeakRcpTrqLim : Outport  Port=4
  wires:
  Rate Limiter Dynamic/1 -> Nm_MotContiDrvTrqLim/1
  w_DisChrgPwrAvail10/1 -> Gain1/1
  Divide/1 -> MinMax/1
  Constant1/1 -> Divide/3, Divide1/3
  Gain1/1 -> Divide/1
  Sum/1 -> MinMax/2
  Nm_Mot1ContiDrvTrqLim/1 -> Sum/1
  Nm_Mot2ContiDrvTrqLim/1 -> Sum/2
  w_DisChrgPwrAvail2/1 -> Gain2/1
  w_ChrgPwrAvail10/1 -> Gain3/1
  speed_to_rev/1(rpm_ActRev) -> Divide3/2, Divide2/2, Divide1/2, Divide/2
  Divide1/1 -> MinMax1/1
  Gain2/1 -> Divide1/1
  Sum4/1 -> MinMax1/2
  Divide2/1 -> MinMax2/1
  Gain3/1 -> Divide2/1
  Sum5/1 -> Abs5/1
  Divide3/1 -> MinMax3/1
  Gain4/1 -> Divide3/1
  Sum6/1 -> Abs6/1
  Nm_Mot1PeakDrvTrqLim/1 -> Sum4/1
  _Nm_Mot2PeakDrvTrqLim/1 -> Sum4/2
  Nm_Mot1PeakRcpTrqLim/1 -> Sum6/1
  Nm_Mot2PeakRcpTrqLim/1 -> Sum6/2
  Nm_Mot1ContiRcpTrqLim/1 -> Sum5/1
  Nm_Mot2ContiRcpTrqLim/1 -> Sum5/2
  w_ChrgPwrAvail2/1 -> Gain4/1
  MinMax/1 -> Rate Limiter Dynamic/2
  Rate Limiter Dynamic1/1 -> Nm_MotPeakDrvTrqLim/1
  MinMax1/1 -> Rate Limiter Dynamic1/2
  Rate Limiter Dynamic2/1 -> Gain5/1
  MinMax2/1 -> Rate Limiter Dynamic2/2
  Rate Limiter Dynamic3/1 -> Gain6/1
  MinMax3/1 -> Rate Limiter Dynamic3/2
  rpm_MCU1MotCtrlActRev/1 -> speed_to_rev/1(rpm_MCU1MotCtrlActRev)
  rpm_MCU2MotCtrlActRev/1 -> speed_to_rev/2(rpm_MCU1TMSpd)
  kmph_VehLgtSpd/1 -> speed_to_rev/3(rpm_MCU2TMSpd)
  Abs5/1 -> MinMax2/2
  Abs6/1 -> MinMax3/2
  Constant3/1 -> Divide2/3, Divide3/3
  Constant2/1 -> Rate Limiter Dynamic/1, Rate Limiter Dynamic1/1
  Constant4/1 -> Rate Limiter Dynamic/3, Rate Limiter Dynamic1/3
  Constant5/1 -> Rate Limiter Dynamic2/1, Rate Limiter Dynamic3/1
  Constant6/1 -> Rate Limiter Dynamic2/3, Rate Limiter Dynamic3/3
  Gain5/1 -> Nm_MotContiRcpTrqLim/1
  Gain6/1 -> Nm_MotPeakRcpTrqLim/1

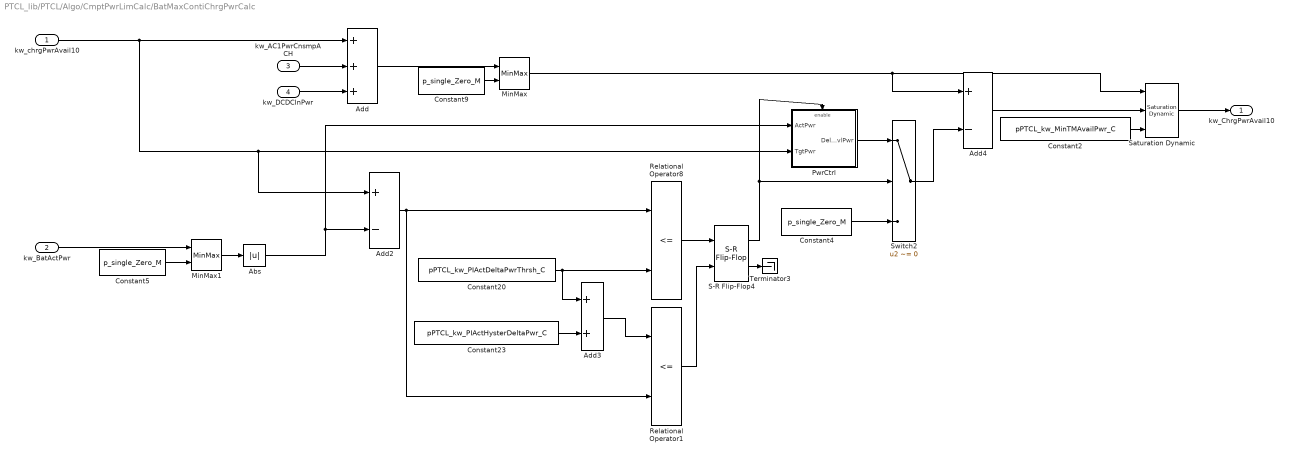
== system PTCL_lib/PTCL/Algo/CmptPwrLimCalc/BatMaxContiChrgPwrCalc ==
  kw_chrgPwrAvail10 : Inport
  kw_BatActPwr : Inport  Port=2
  kw_AC1PwrCnsmpACH : Inport  Port=3
  kw_DCDCInPwr : Inport  Port=4
  Abs : Abs  SaturateOnIntegerOverflow=on
      mask Display: patch([0 1 1 1 .75], [1 1 0 .75 1], [0 1 0]);
  Add : Sum  Inputs=+++  SaturateOnIntegerOverflow=on  InputSameDT=on  OutDataTypeStr=Inherit: Same as first input
      mask Display: patch([0 1 1 1 .75], [1 1 0 .75 1], [0 1 0]);
  Add2 : Sum  Inputs=+-  SaturateOnIntegerOverflow=on  InputSameDT=on  OutDataTypeStr=Inherit: Same as first input
      mask Display: patch([0 1 1 1 .75], [1 1 0 .75 1], [0 1 0]);
  Add3 : Sum  SaturateOnIntegerOverflow=on  InputSameDT=on  OutDataTypeStr=Inherit: Same as first input
      mask Display: patch([0 1 1 1 .75], [1 1 0 .75 1], [0 1 0]);
  Add4 : Sum  Inputs=+-  SaturateOnIntegerOverflow=on  InputSameDT=on  OutDataTypeStr=Inherit: Same as first input
      mask Display: patch([0 1 1 1 .75], [1 1 0 .75 1], [0 1 0]);
  Constant2 : Constant  Value=pPTCL_kw_MinTMAvailPwr_C
      mask Display: patch([0 1 1 1 .75], [1 1 0 .75 1], [0 1 0]);
  Constant20 : Constant  Value=pPTCL_kw_PIActDeltaPwrThrsh_C
      mask Display: patch([0 1 1 1 .75], [1 1 0 .75 1], [0 1 0]);
  Constant23 : Constant  Value=pPTCL_kw_PIActHysterDeltaPwr_C
      mask Display: patch([0 1 1 1 .75], [1 1 0 .75 1], [0 1 0]);
  Constant4 : Constant  Value=p_single_Zero_M
      mask Display: patch([0 1 1 1 .75], [1 1 0 .75 1], [0 1 0]);
  Constant5 : Constant  Value=p_single_Zero_M
      mask Display: patch([0 1 1 1 .75], [1 1 0 .75 1], [0 1 0]);
  Constant9 : Constant  Value=p_single_Zero_M
      mask Display: patch([0 1 1 1 .75], [1 1 0 .75 1], [0 1 0]);
  MinMax : BaseOperationLib_Browser/Math Operations Changed/MinMax  Function=max  Inputs=2  InputSameDT=on  OutMin=[]  OutMax=[]  OutDataType=fixdt(1,16,0)  OutScaling=[]  SaturateOnIntegerOverflow=on
  MinMax1 : BaseOperationLib_Browser/Math Operations Changed/MinMax  Function=min  Inputs=2  InputSameDT=on  OutMin=[]  OutMax=[]  OutDataType=fixdt(1,16,0)  OutScaling=[]  SaturateOnIntegerOverflow=on
  PwrCtrl : Subsystem
  Relational Operator1 : RelationalOperator  Operator=<=  LogicOutDataTypeMode=Specify via dialog  LogicDataType=PDT_Bool  OutDataTypeStr=PDT_Bool  InputSameDT=on
      mask Display: patch([0 1 1 1 .75], [1 1 0 .75 1], [0 1 0]);
  Relational Operator8 : RelationalOperator  Operator=<=  LogicOutDataTypeMode=Specify via dialog  LogicDataType=PDT_Bool  OutDataTypeStr=PDT_Bool  InputSameDT=on
      mask Display: patch([0 1 1 1 .75], [1 1 0 .75 1], [0 1 0]);
  S-R Flip-Flop4 : BaseOperationLib_Browser/Others Unchanged/S-R Flip-Flop  SystemSampleTime=-1  initial_condition=0
  Saturation Dynamic : BaseOperationLib_Browser/Discontinuities Unchanged/Saturation Dynamic  SystemSampleTime=-1  OutMin=[]  OutMax=[]  OutDataTypeStr=Inherit: Same as second input  OutDataType=fixdt(1, 16)  OutScaling=2^-10  DoSatur=on
  Switch2 : Switch  Criteria=u2 ~= 0  SaturateOnIntegerOverflow=on  InputSameDT=on
      mask Display: patch([0 1 1 1 .75], [1 1 0 .75 1], [0 1 0]);
  Terminator3 : Terminator
  kw_ChrgPwrAvail10 : Outport  OutDataType=fixdt(1, 16)  OutScaling=2^0
  wires:
  kw_BatActPwr/1 -> MinMax1/1
  MinMax1/1 -> Abs/1
  Constant5/1 -> MinMax1/2
  Abs/1 -> Add2/2, PwrCtrl/1(ActPwr)
  Add/1 -> MinMax/1
  Constant9/1 -> MinMax/2
  Constant2/1 -> Saturation Dynamic/3
  kw_chrgPwrAvail10/1 -> Add/1, Add2/1, PwrCtrl/2(TgtPwr)
  S-R Flip-Flop4/2 -> Terminator3/1
  Add2/1 -> Relational Operator8/1, Relational Operator1/2
  Constant20/1 -> Relational Operator8/2, Add3/1
  Constant23/1 -> Add3/2
  Add3/1 -> Relational Operator1/1
  Relational Operator8/1 -> S-R Flip-Flop4/1
  Relational Operator1/1 -> S-R Flip-Flop4/2
  S-R Flip-Flop4/1 -> Switch2/2, PwrCtrl/Enable
  Constant4/1 -> Switch2/3
  Switch2/1 -> Add4/2
  PwrCtrl/1(DeltaEMAvlPwr) -> Switch2/1
  Add4/1 -> Saturation Dynamic/2
  MinMax/1 -> Add4/1, Saturation Dynamic/1
  kw_AC1PwrCnsmpACH/1 -> Add/2
  kw_DCDCInPwr/1 -> Add/3
  Saturation Dynamic/1 -> kw_ChrgPwrAvail10/1

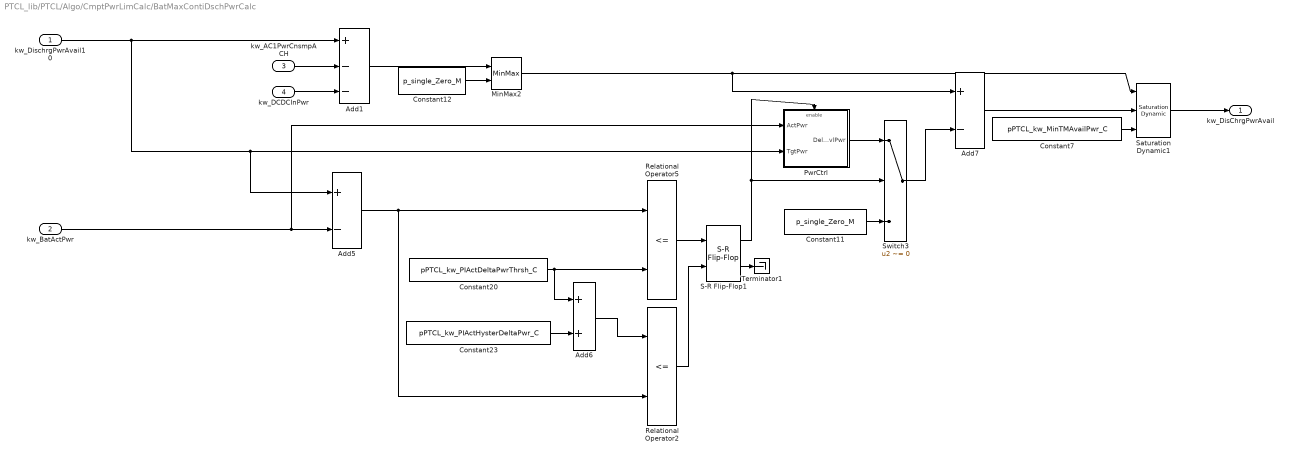
== system PTCL_lib/PTCL/Algo/CmptPwrLimCalc/BatMaxContiDschPwrCalc ==
  kw_DischrgPwrAvail10 : Inport
  kw_BatActPwr : Inport  Port=2
  kw_AC1PwrCnsmpACH : Inport  Port=3
  kw_DCDCInPwr : Inport  Port=4
  Add1 : Sum  Inputs=+--  SaturateOnIntegerOverflow=on  InputSameDT=on  OutDataTypeStr=Inherit: Same as first input
      mask Display: patch([0 1 1 1 .75], [1 1 0 .75 1], [0 1 0]);
  Add5 : Sum  Inputs=+-  SaturateOnIntegerOverflow=on  InputSameDT=on  OutDataTypeStr=Inherit: Same as first input
      mask Display: patch([0 1 1 1 .75], [1 1 0 .75 1], [0 1 0]);
  Add6 : Sum  SaturateOnIntegerOverflow=on  InputSameDT=on  OutDataTypeStr=Inherit: Same as first input
      mask Display: patch([0 1 1 1 .75], [1 1 0 .75 1], [0 1 0]);
  Add7 : Sum  Inputs=+-  SaturateOnIntegerOverflow=on  InputSameDT=on  OutDataTypeStr=Inherit: Same as first input
      mask Display: patch([0 1 1 1 .75], [1 1 0 .75 1], [0 1 0]);
  Constant11 : Constant  Value=p_single_Zero_M
      mask Display: patch([0 1 1 1 .75], [1 1 0 .75 1], [0 1 0]);
  Constant12 : Constant  Value=p_single_Zero_M
      mask Display: patch([0 1 1 1 .75], [1 1 0 .75 1], [0 1 0]);
  Constant20 : Constant  Value=pPTCL_kw_PIActDeltaPwrThrsh_C
      mask Display: patch([0 1 1 1 .75], [1 1 0 .75 1], [0 1 0]);
  Constant23 : Constant  Value=pPTCL_kw_PIActHysterDeltaPwr_C
      mask Display: patch([0 1 1 1 .75], [1 1 0 .75 1], [0 1 0]);
  Constant7 : Constant  Value=pPTCL_kw_MinTMAvailPwr_C
      mask Display: patch([0 1 1 1 .75], [1 1 0 .75 1], [0 1 0]);
  MinMax2 : BaseOperationLib_Browser/Math Operations Changed/MinMax  Function=max  Inputs=2  InputSameDT=on  OutMin=[]  OutMax=[]  OutDataType=fixdt(1,16,0)  OutScaling=[]  SaturateOnIntegerOverflow=on
  PwrCtrl : Subsystem
  Relational Operator2 : RelationalOperator  Operator=<=  LogicOutDataTypeMode=Specify via dialog  LogicDataType=PDT_Bool  OutDataTypeStr=PDT_Bool  InputSameDT=on
      mask Display: patch([0 1 1 1 .75], [1 1 0 .75 1], [0 1 0]);
  Relational Operator5 : RelationalOperator  Operator=<=  LogicOutDataTypeMode=Specify via dialog  LogicDataType=PDT_Bool  OutDataTypeStr=PDT_Bool  InputSameDT=on
      mask Display: patch([0 1 1 1 .75], [1 1 0 .75 1], [0 1 0]);
  S-R Flip-Flop1 : BaseOperationLib_Browser/Others Unchanged/S-R Flip-Flop  SystemSampleTime=-1  initial_condition=0
  Saturation Dynamic1 : BaseOperationLib_Browser/Discontinuities Unchanged/Saturation Dynamic  SystemSampleTime=-1  OutMin=[]  OutMax=[]  OutDataTypeStr=Inherit: Same as second input  OutDataType=fixdt(1, 16)  OutScaling=2^-10  DoSatur=on
  Switch3 : Switch  Criteria=u2 ~= 0  SaturateOnIntegerOverflow=on  InputSameDT=on
      mask Display: patch([0 1 1 1 .75], [1 1 0 .75 1], [0 1 0]);
  Terminator1 : Terminator
  kw_DisChrgPwrAvail : Outport  OutDataType=fixdt(1, 16)  OutScaling=2^0
  wires:
  Add1/1 -> MinMax2/1
  Constant12/1 -> MinMax2/2
  Constant7/1 -> Saturation Dynamic1/3
  kw_DischrgPwrAvail10/1 -> Add1/1, Add5/1, PwrCtrl/2(TgtPwr)
  S-R Flip-Flop1/2 -> Terminator1/1
  Add5/1 -> Relational Operator5/1, Relational Operator2/2
  Constant20/1 -> Relational Operator5/2, Add6/1
  Constant23/1 -> Add6/2
  Add6/1 -> Relational Operator2/1
  Relational Operator5/1 -> S-R Flip-Flop1/1
  Relational Operator2/1 -> S-R Flip-Flop1/2
  S-R Flip-Flop1/1 -> Switch3/2, PwrCtrl/Enable
  Constant11/1 -> Switch3/3
  Switch3/1 -> Add7/2
  PwrCtrl/1(DeltaEMAvlPwr) -> Switch3/1
  Add7/1 -> Saturation Dynamic1/2
  MinMax2/1 -> Add7/1, Saturation Dynamic1/1
  kw_BatActPwr/1 -> Add5/2, PwrCtrl/1(ActPwr)
  kw_AC1PwrCnsmpACH/1 -> Add1/2
  kw_DCDCInPwr/1 -> Add1/3
  Saturation Dynamic1/1 -> kw_DisChrgPwrAvail/1

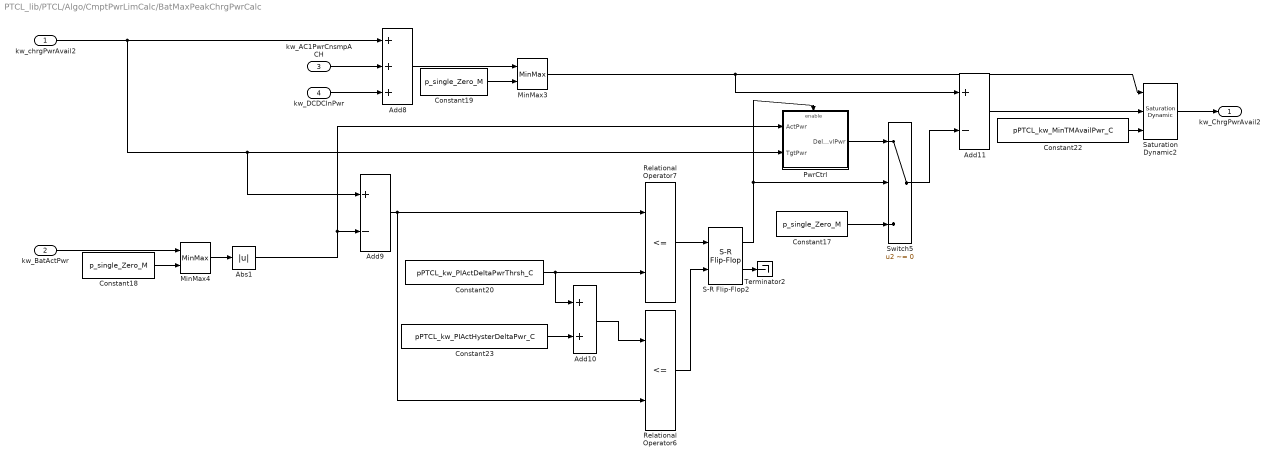
== system PTCL_lib/PTCL/Algo/CmptPwrLimCalc/BatMaxPeakChrgPwrCalc ==
  kw_chrgPwrAvail2 : Inport
  kw_BatActPwr : Inport  Port=2
  kw_AC1PwrCnsmpACH : Inport  Port=3
  kw_DCDCInPwr : Inport  Port=4
  Abs1 : Abs  SaturateOnIntegerOverflow=on
      mask Display: patch([0 1 1 1 .75], [1 1 0 .75 1], [0 1 0]);
  Add10 : Sum  SaturateOnIntegerOverflow=on  InputSameDT=on  OutDataTypeStr=Inherit: Same as first input
      mask Display: patch([0 1 1 1 .75], [1 1 0 .75 1], [0 1 0]);
  Add11 : Sum  Inputs=+-  SaturateOnIntegerOverflow=on  InputSameDT=on  OutDataTypeStr=Inherit: Same as first input
      mask Display: patch([0 1 1 1 .75], [1 1 0 .75 1], [0 1 0]);
  Add8 : Sum  Inputs=+++  SaturateOnIntegerOverflow=on  InputSameDT=on  OutDataTypeStr=Inherit: Same as first input
      mask Display: patch([0 1 1 1 .75], [1 1 0 .75 1], [0 1 0]);
  Add9 : Sum  Inputs=+-  SaturateOnIntegerOverflow=on  InputSameDT=on  OutDataTypeStr=Inherit: Same as first input
      mask Display: patch([0 1 1 1 .75], [1 1 0 .75 1], [0 1 0]);
  Constant17 : Constant  Value=p_single_Zero_M
      mask Display: patch([0 1 1 1 .75], [1 1 0 .75 1], [0 1 0]);
  Constant18 : Constant  Value=p_single_Zero_M
      mask Display: patch([0 1 1 1 .75], [1 1 0 .75 1], [0 1 0]);
  Constant19 : Constant  Value=p_single_Zero_M
      mask Display: patch([0 1 1 1 .75], [1 1 0 .75 1], [0 1 0]);
  Constant20 : Constant  Value=pPTCL_kw_PIActDeltaPwrThrsh_C
      mask Display: patch([0 1 1 1 .75], [1 1 0 .75 1], [0 1 0]);
  Constant22 : Constant  Value=pPTCL_kw_MinTMAvailPwr_C
      mask Display: patch([0 1 1 1 .75], [1 1 0 .75 1], [0 1 0]);
  Constant23 : Constant  Value=pPTCL_kw_PIActHysterDeltaPwr_C
      mask Display: patch([0 1 1 1 .75], [1 1 0 .75 1], [0 1 0]);
  MinMax3 : BaseOperationLib_Browser/Math Operations Changed/MinMax  Function=max  Inputs=2  InputSameDT=on  OutMin=[]  OutMax=[]  OutDataType=fixdt(1,16,0)  OutScaling=[]  SaturateOnIntegerOverflow=on
  MinMax4 : BaseOperationLib_Browser/Math Operations Changed/MinMax  Function=min  Inputs=2  InputSameDT=on  OutMin=[]  OutMax=[]  OutDataType=fixdt(1,16,0)  OutScaling=[]  SaturateOnIntegerOverflow=on
  PwrCtrl : Subsystem
  Relational Operator6 : RelationalOperator  Operator=<=  LogicOutDataTypeMode=Specify via dialog  LogicDataType=PDT_Bool  OutDataTypeStr=PDT_Bool  InputSameDT=on
      mask Display: patch([0 1 1 1 .75], [1 1 0 .75 1], [0 1 0]);
  Relational Operator7 : RelationalOperator  Operator=<=  LogicOutDataTypeMode=Specify via dialog  LogicDataType=PDT_Bool  OutDataTypeStr=PDT_Bool  InputSameDT=on
      mask Display: patch([0 1 1 1 .75], [1 1 0 .75 1], [0 1 0]);
  S-R Flip-Flop2 : BaseOperationLib_Browser/Others Unchanged/S-R Flip-Flop  SystemSampleTime=-1  initial_condition=0
  Saturation Dynamic2 : BaseOperationLib_Browser/Discontinuities Unchanged/Saturation Dynamic  SystemSampleTime=-1  OutMin=[]  OutMax=[]  OutDataTypeStr=Inherit: Same as second input  OutDataType=fixdt(1, 16)  OutScaling=2^-10  DoSatur=on
  Switch5 : Switch  Criteria=u2 ~= 0  SaturateOnIntegerOverflow=on  InputSameDT=on
      mask Display: patch([0 1 1 1 .75], [1 1 0 .75 1], [0 1 0]);
  Terminator2 : Terminator
  kw_ChrgPwrAvail2 : Outport  OutDataType=fixdt(1, 16)  OutScaling=2^0
  wires:
  MinMax3/1 -> Saturation Dynamic2/1, Add11/1
  Add11/1 -> Saturation Dynamic2/2
  PwrCtrl/1(DeltaEMAvlPwr) -> Switch5/1
  Switch5/1 -> Add11/2
  Constant17/1 -> Switch5/3
  S-R Flip-Flop2/1 -> Switch5/2, PwrCtrl/Enable
  Relational Operator6/1 -> S-R Flip-Flop2/2
  Relational Operator7/1 -> S-R Flip-Flop2/1
  Add10/1 -> Relational Operator6/1
  Constant23/1 -> Add10/2
  Constant20/1 -> Add10/1, Relational Operator7/2
  Add9/1 -> Relational Operator6/2, Relational Operator7/1
  S-R Flip-Flop2/2 -> Terminator2/1
  kw_chrgPwrAvail2/1 -> Add8/1, Add9/1, PwrCtrl/2(TgtPwr)
  Constant22/1 -> Saturation Dynamic2/3
  Constant19/1 -> MinMax3/2
  Add8/1 -> MinMax3/1
  Abs1/1 -> Add9/2, PwrCtrl/1(ActPwr)
  Constant18/1 -> MinMax4/2
  MinMax4/1 -> Abs1/1
  kw_BatActPwr/1 -> MinMax4/1
  kw_AC1PwrCnsmpACH/1 -> Add8/2
  kw_DCDCInPwr/1 -> Add8/3
  Saturation Dynamic2/1 -> kw_ChrgPwrAvail2/1

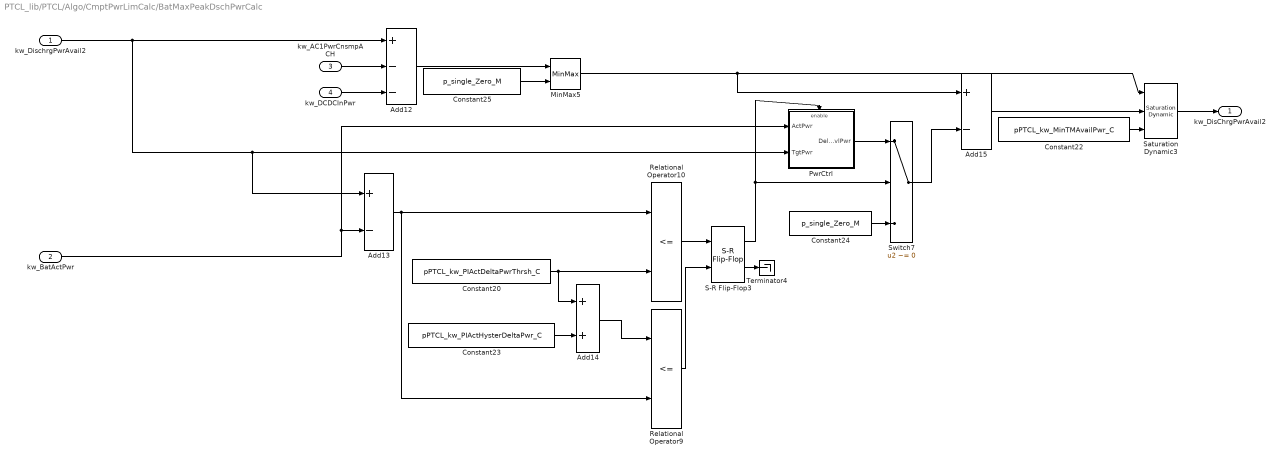
== system PTCL_lib/PTCL/Algo/CmptPwrLimCalc/BatMaxPeakDschPwrCalc ==
  kw_DischrgPwrAvail2 : Inport
  kw_BatActPwr : Inport  Port=2
  kw_AC1PwrCnsmpACH : Inport  Port=3
  kw_DCDCInPwr : Inport  Port=4
  Add12 : Sum  Inputs=+--  SaturateOnIntegerOverflow=on  InputSameDT=on  OutDataTypeStr=Inherit: Same as first input
      mask Display: patch([0 1 1 1 .75], [1 1 0 .75 1], [0 1 0]);
  Add13 : Sum  Inputs=+-  SaturateOnIntegerOverflow=on  InputSameDT=on  OutDataTypeStr=Inherit: Same as first input
      mask Display: patch([0 1 1 1 .75], [1 1 0 .75 1], [0 1 0]);
  Add14 : Sum  SaturateOnIntegerOverflow=on  InputSameDT=on  OutDataTypeStr=Inherit: Same as first input
      mask Display: patch([0 1 1 1 .75], [1 1 0 .75 1], [0 1 0]);
  Add15 : Sum  Inputs=+-  SaturateOnIntegerOverflow=on  InputSameDT=on  OutDataTypeStr=Inherit: Same as first input
      mask Display: patch([0 1 1 1 .75], [1 1 0 .75 1], [0 1 0]);
  Constant20 : Constant  Value=pPTCL_kw_PIActDeltaPwrThrsh_C
      mask Display: patch([0 1 1 1 .75], [1 1 0 .75 1], [0 1 0]);
  Constant22 : Constant  Value=pPTCL_kw_MinTMAvailPwr_C
      mask Display: patch([0 1 1 1 .75], [1 1 0 .75 1], [0 1 0]);
  Constant23 : Constant  Value=pPTCL_kw_PIActHysterDeltaPwr_C
      mask Display: patch([0 1 1 1 .75], [1 1 0 .75 1], [0 1 0]);
  Constant24 : Constant  Value=p_single_Zero_M
      mask Display: patch([0 1 1 1 .75], [1 1 0 .75 1], [0 1 0]);
  Constant25 : Constant  Value=p_single_Zero_M
      mask Display: patch([0 1 1 1 .75], [1 1 0 .75 1], [0 1 0]);
  MinMax5 : BaseOperationLib_Browser/Math Operations Changed/MinMax  Function=max  Inputs=2  InputSameDT=on  OutMin=[]  OutMax=[]  OutDataType=fixdt(1,16,0)  OutScaling=[]  SaturateOnIntegerOverflow=on
  PwrCtrl : Subsystem
  Relational Operator10 : RelationalOperator  Operator=<=  LogicOutDataTypeMode=Specify via dialog  LogicDataType=PDT_Bool  OutDataTypeStr=PDT_Bool  InputSameDT=on
      mask Display: patch([0 1 1 1 .75], [1 1 0 .75 1], [0 1 0]);
  Relational Operator9 : RelationalOperator  Operator=<=  LogicOutDataTypeMode=Specify via dialog  LogicDataType=PDT_Bool  OutDataTypeStr=PDT_Bool  InputSameDT=on
      mask Display: patch([0 1 1 1 .75], [1 1 0 .75 1], [0 1 0]);
  S-R Flip-Flop3 : BaseOperationLib_Browser/Others Unchanged/S-R Flip-Flop  SystemSampleTime=-1  initial_condition=0
  Saturation Dynamic3 : BaseOperationLib_Browser/Discontinuities Unchanged/Saturation Dynamic  SystemSampleTime=-1  OutMin=[]  OutMax=[]  OutDataTypeStr=Inherit: Same as second input  OutDataType=fixdt(1, 16)  OutScaling=2^-10  DoSatur=on
  Switch7 : Switch  Criteria=u2 ~= 0  SaturateOnIntegerOverflow=on  InputSameDT=on
      mask Display: patch([0 1 1 1 .75], [1 1 0 .75 1], [0 1 0]);
  Terminator4 : Terminator
  kw_DisChrgPwrAvail2 : Outport  OutDataType=fixdt(1, 16)  OutScaling=2^0
  wires:
  MinMax5/1 -> Saturation Dynamic3/1, Add15/1
  Add15/1 -> Saturation Dynamic3/2
  PwrCtrl/1(DeltaEMAvlPwr) -> Switch7/1
  Switch7/1 -> Add15/2
  Constant24/1 -> Switch7/3
  S-R Flip-Flop3/1 -> Switch7/2, PwrCtrl/Enable
  Relational Operator9/1 -> S-R Flip-Flop3/2
  Relational Operator10/1 -> S-R Flip-Flop3/1
  Add14/1 -> Relational Operator9/1
  Constant23/1 -> Add14/2
  Constant20/1 -> Add14/1, Relational Operator10/2
  Add13/1 -> Relational Operator9/2, Relational Operator10/1
  kw_BatActPwr/1 -> Add13/2, PwrCtrl/1(ActPwr)
  S-R Flip-Flop3/2 -> Terminator4/1
  kw_DischrgPwrAvail2/1 -> Add12/1, Add13/1, PwrCtrl/2(TgtPwr)
  Constant22/1 -> Saturation Dynamic3/3
  Constant25/1 -> MinMax5/2
  Add12/1 -> MinMax5/1
  kw_AC1PwrCnsmpACH/1 -> Add12/2
  kw_DCDCInPwr/1 -> Add12/3
  Saturation Dynamic3/1 -> kw_DisChrgPwrAvail2/1
